simulink model "close_circuit"  (R2022a)
settings: Solver=ode45  StartTime=0.0  StopTime=0.002  MaxStep=1e-8  RelTol=1e-3
undefined symbols (not defined in the file or in its folder): plecs
libraries: simulink x1
settings Model: Creator=LIU  LastModifiedBy=LIU

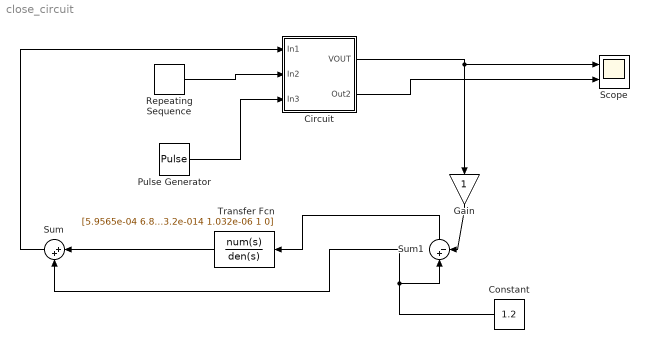
== system close_circuit ==
  Circuit : Subsystem  LoadFcn=plecs('sl', 200);  InitFcn=plecs('sl', 214);  StartFcn=plecs('sl', 208);  StopFcn=plecs('sl', 209);  mask(PlecsCircuit){PLECSData=<binary blob, 3264 chars, not shown>}
      mask prompts: PLECSData "PLECS Data (Do not delete or modify!)"
      mask init:
      | % PLACE CUSTOM INITIALIZATIONS ABOVE
      | % DO NOT REMOVE
      | plecs('sl', 215);
      | % DO NOT REMOVE
      settings: CopyFcn=plecs('sl', 203);  DeleteFcn=plecs('sl', 205);  UndoDeleteFcn=plecs('sl', 206);  PreSaveFcn=plecs('sl', 211);  PostSaveFcn=plecs('sl', 201);  NameChangeFcn=plecs('sl', 210);  DestroyFcn=plecs('sl', 207);  PreCopyFcn=plecs('sl', 216);  OpenFcn=plecs('sl', 202);  ErrorFcn=plerrorfcn
      mask Help: web(['file:///' fullfile(plecsdoc, 'creatingacircuit.html')])
      mask Display: disp('PLECS\nCircuit')
  Constant : Constant  Value=1.2
  Gain : Gain
  Pulse Generator : DiscretePulseGenerator  PulseType=Time based  Period=0.001  PulseWidth=50
  Repeating Sequence : simulink/Sources/Repeating Sequence  rep_seq_t=[0 2e-6]  rep_seq_y=[0 3]
  Scope : Scope  NumInputPorts=2
  Sum : Sum  Inputs=|++
  Sum1 : Sum  Inputs=|+-
  Transfer Fcn : TransferFcn  Numerator=[5.9565e-04 6.859 9025]  Denominator=[3.2e-014 1.032e-06 1 0]
  wires:
  Transfer Fcn/1 -> Sum/1
  Sum1/1 -> Transfer Fcn/1
  Sum/1 -> Circuit/1(In1)
  Circuit/2(Out2) -> Scope/2
  Circuit/1(VOUT) -> Scope/1, Gain/1
  Pulse Generator/1 -> Circuit/3(In3)
  Repeating Sequence/1 -> Circuit/2(In2)
  Constant/1 -> Sum/2, Sum1/1
  Gain/1 -> Sum1/2

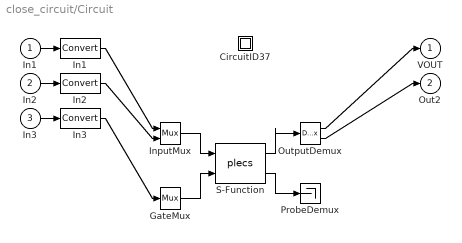
== system close_circuit/Circuit ==
  In1 : Inport  PortDimensions=1
  In2 : Inport  Port=2  PortDimensions=1
  In3 : Inport  Port=3  PortDimensions=1
  " CircuitID37 " : Subsystem
  " GateMux " : Mux  Inputs=[ 1 ]
  " In1 " : DataTypeConversion
  " In2 " : DataTypeConversion
  " In3 " : DataTypeConversion
  " InputMux " : Mux  Inputs=[ 1 1 ]
  " OutputDemux " : Demux  Outputs=[ 1 1 ]
  " ProbeDemux " : Terminator
  " S-Function " : S-Function  FunctionName=plecs  SFunctionDeploymentMode=off  EnableBusSupport=off
  VOUT : Outport  PortDimensions=1
  Out2 : Outport  Port=2  PortDimensions=1
  wires:
  " S-Function "/1 -> " OutputDemux "/1
  " InputMux "/1 -> " S-Function "/1
  " GateMux "/1 -> " S-Function "/2
  " S-Function "/2 -> " ProbeDemux "/1
  In1/1 -> " In1 "/1
  " In1 "/1 -> " InputMux "/1
  In2/1 -> " In2 "/1
  " In2 "/1 -> " InputMux "/2
  In3/1 -> " In3 "/1
  " In3 "/1 -> " GateMux "/1
  " OutputDemux "/1 -> VOUT/1
  " OutputDemux "/2 -> Out2/1

== system close_circuit/Circuit/ CircuitID37  ==
